simulink model "EdgeDetection"  (R2021a)
settings: Solver=VariableStepAuto  StartTime=0.0  StopTime=Ts_480p*2  RelTol=1e-3
InitFcn:
  | Ts = 1e-3;
  | Ts_240p = 402*324*Ts;
  | Ts_480p = 525*800*Ts;
undefined symbols (not defined in the file): gray, Rec, SDTV
libraries: hdlsllib x7, simulink x5, visionhdlio x2, visionhdlconversions x1, dspvision x1
settings Model: Creator=user  LastModifiedBy=user
settings OptimizationCC: BlockReduction=off  ConditionallyExecuteInputs=off  DefaultParameterBehavior=Inlined
settings DebuggingCC: AlgebraicLoopMsg=error
settings HardwareCC: ProdBitPerPointer=32  ProdBitPerSizeT=32  ProdBitPerPtrDiffT=32  ProdLargestAtomicFloat=None  ProdIntDivRoundTo=Undefined  ProdEndianess=Unspecified  ProdWordSize=32  ProdHWDeviceType=ASIC/FPGA->ASIC/FPGA  TargetBitPerPointer=64  TargetBitPerSizeT=64  TargetBitPerPtrDiffT=64  TargetLongLongMode=on  TargetIntDivRoundTo=Zero  TargetEndianess=LittleEndian  TargetWordSize=64  TargetHWDeviceType=Custom Processor->MATLAB Host Computer  ProdEqTarget=off

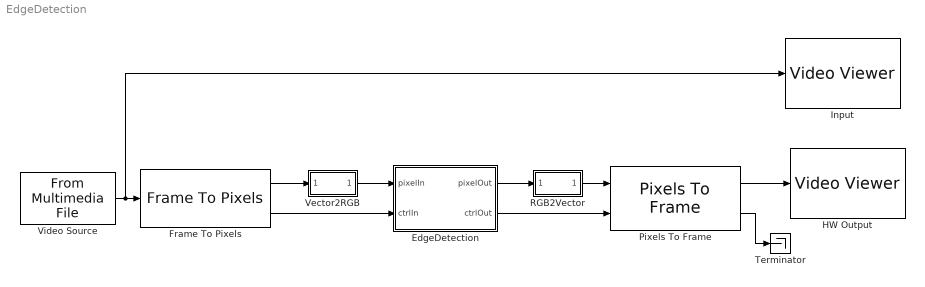
== system EdgeDetection ==
  EdgeDetection : Subsystem  TreatAsAtomicUnit=on
  Frame To Pixels : visionhdlio/Frame To Pixels  NumComponents=3  NumPixels=1  VideoFormat=480p  ActivePixelsPerLine=32  ActiveVideoLines=18  TotalPixelsPerLine=42  TotalVideoLines=28  StartingActiveLine=6  FrontPorch=5  SampleTime=0
      settings: SourceProductBaseCode=VT
  HW Output : VideoViewer  colormapValue=gray(256)  FigPos=[237 717 588 436]
  Input : VideoViewer  colormapValue=gray(256)  FigPos=[896 724 588 436]
  Pixels To Frame : visionhdlio/Pixels To Frame  NumComponents=3  NumPixels=1  VideoFormat=480p  ActivePixelsPerLine=32  ActiveVideoLines=18  TotalPixelsPerLine=42  TotalVideoLines=28
      settings: SourceProductBaseCode=VT
  RGB2Vector : Subsystem
  Terminator : Terminator
  Vector2RGB : Subsystem
  Video Source : dspvision/From Multimedia File  inputFilename=D:\Work\XilFPGAdev\Custom_IP_Cores\MathworksHDLCoder\testImages\engine_480p.bmp  readRange=[1 Inf]  loop=on  numPlays=inf  outputStreams=Video only  videoDataType=uint8  audioDataType=int16  inheritSampleTime=off  userDefinedSampleTime=Ts_480p  noAudioOutput=off  isIntensityVideo=off  fourcc=RGB  colorVideoFormat=One multidimensional signal  outputEOF=off  dataOrg=Column-major  audioFrameSize=1024  computeAudioFrameSize=off  outSamplingMode=Sample based
  wires:
  Vector2RGB/1(RGB) -> EdgeDetection/1(pixelIn)
  RGB2Vector/1(RGBVector) -> Pixels To Frame/1
  Frame To Pixels/1 -> Vector2RGB/1(RGBVector)
  Frame To Pixels/2 -> EdgeDetection/2(ctrlIn)
  Pixels To Frame/1 -> HW Output/1
  Pixels To Frame/2 -> Terminator/1
  Video Source/1 -> Input/1, Frame To Pixels/1
  EdgeDetection/1(pixelOut) -> RGB2Vector/1(RGB)
  EdgeDetection/2(ctrlOut) -> Pixels To Frame/2

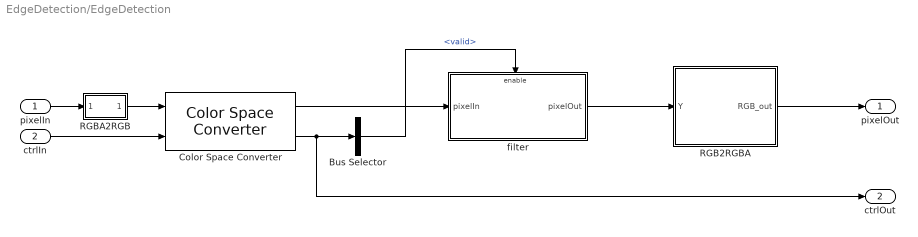
== system EdgeDetection/EdgeDetection ==
  pixelIn : Inport
  ctrlIn : Inport  Port=2
  Bus Selector : BusSelector  OutputSignals=valid
  Color Space Converter : visionhdlconversions/Color Space Converter  Conversion=RGB to intensity  ConversionStandard=Rec. 601 (SDTV)  ScanningStandard=1250/50/2:1  SimulateUsing=Code generation
      settings: SourceProductBaseCode=VT
  RGB2RGBA : MATLAB Function  TreatAsAtomicUnit=on
  RGBA2RGB : Subsystem
  filter : Subsystem
  pixelOut : Outport
  ctrlOut : Outport  Port=2  VectorParamsAs1DForOutWhenUnconnected=off
  wires:
  ctrlIn/1 -> Color Space Converter/2
  pixelIn/1 -> RGBA2RGB/1(RGBA)
  Color Space Converter/2 -> Bus Selector/1, ctrlOut/1
  RGBA2RGB/1(RGB) -> Color Space Converter/1
  RGB2RGBA/1(RGB_out) -> pixelOut/1
  Color Space Converter/1 -> filter/1(pixelIn)
  Bus Selector/1 -> filter/Enable  "<valid>"
  filter/1(pixelOut) -> RGB2RGBA/1(Y)

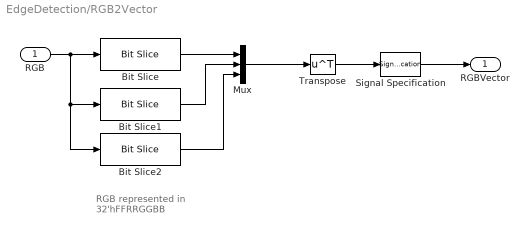
== system EdgeDetection/RGB2Vector ==
  note: RGB represented in
      | 32'hFFRRGGBB
  RGB : Inport
  Bit Slice : hdlsllib/Logic and Bit Operations/Bit Slice  lidx=23  ridx=16
      settings: SourceProductBaseCode=SL
  Bit Slice1 : hdlsllib/Logic and Bit Operations/Bit Slice  lidx=15  ridx=8
      settings: SourceProductBaseCode=SL
  Bit Slice2 : hdlsllib/Logic and Bit Operations/Bit Slice  lidx=7  ridx=0
      settings: SourceProductBaseCode=SL
  Mux : Mux  Inputs=3
  Signal Specification : SignalSpecification
  Transpose : Math  Operator=transpose  SignedPower=on  SaturateOnIntegerOverflow=on
  RGBVector : Outport  VectorParamsAs1DForOutWhenUnconnected=off
  wires:
  Mux/1 -> Transpose/1
  Bit Slice/1 -> Mux/1
  Bit Slice2/1 -> Mux/3
  Bit Slice1/1 -> Mux/2
  RGB/1 -> Bit Slice2/1, Bit Slice1/1, Bit Slice/1
  Transpose/1 -> Signal Specification/1
  Signal Specification/1 -> RGBVector/1

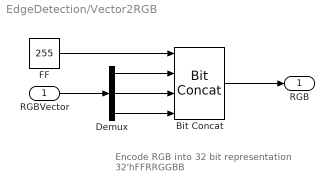
== system EdgeDetection/Vector2RGB ==
  note: Encode RGB into 32 bit representation
      | 32'hFFRRGGBB
  RGBVector : Inport
  Bit Concat : hdlsllib/Logic and Bit Operations/Bit Concat  numInputs=4
  Demux : Demux  Outputs=3
  FF : Constant  Value=255  OutDataTypeStr=uint8  SampleTime=Ts
  RGB : Outport  VectorParamsAs1DForOutWhenUnconnected=off
  wires:
  Bit Concat/1 -> RGB/1
  RGBVector/1 -> Demux/1
  FF/1 -> Bit Concat/1
  Demux/1 -> Bit Concat/2
  Demux/2 -> Bit Concat/3
  Demux/3 -> Bit Concat/4

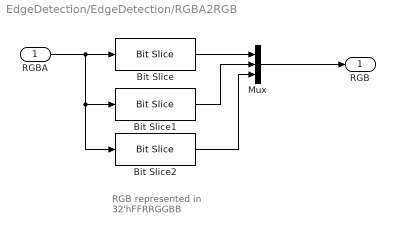
== system EdgeDetection/EdgeDetection/RGBA2RGB ==
  note: RGB represented in
      | 32'hFFRRGGBB
  RGBA : Inport
  Bit Slice : hdlsllib/Logic and Bit Operations/Bit Slice  lidx=23  ridx=16
      settings: SourceProductBaseCode=SL
  Bit Slice1 : hdlsllib/Logic and Bit Operations/Bit Slice  lidx=15  ridx=8
      settings: SourceProductBaseCode=SL
  Bit Slice2 : hdlsllib/Logic and Bit Operations/Bit Slice  lidx=7  ridx=0
      settings: SourceProductBaseCode=SL
  Mux : Mux  Inputs=3
  RGB : Outport  VectorParamsAs1DForOutWhenUnconnected=off
  wires:
  Bit Slice/1 -> Mux/1
  Bit Slice2/1 -> Mux/3
  Bit Slice1/1 -> Mux/2
  RGBA/1 -> Bit Slice2/1, Bit Slice1/1, Bit Slice/1
  Mux/1 -> RGB/1

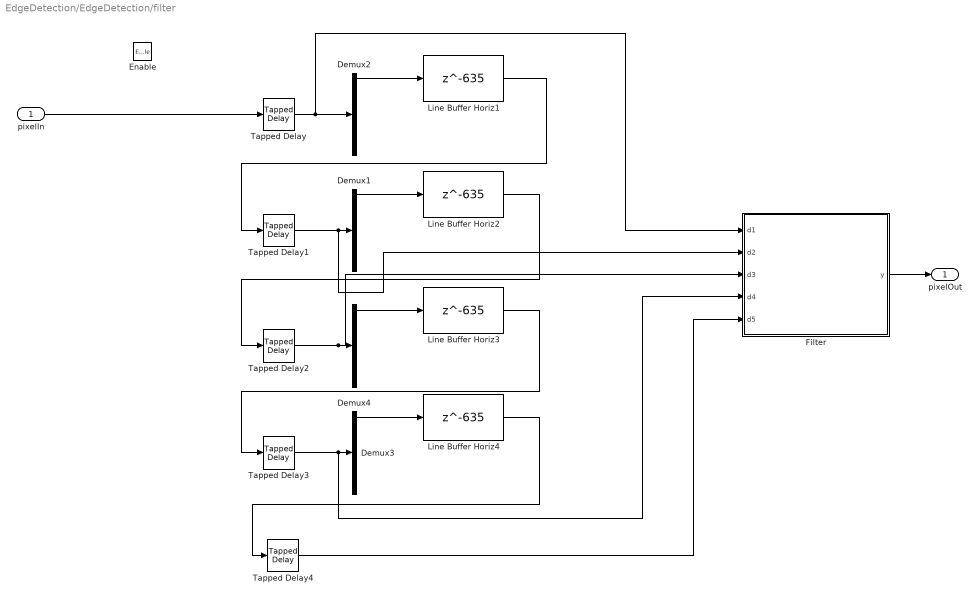
== system EdgeDetection/EdgeDetection/filter ==
  pixelIn : Inport
  Enable : EnablePort
  Demux{1..4} (4 alike) : Demux  Outputs=5
      settings: DisplayOption=none
  Filter : MATLAB Function  TreatAsAtomicUnit=on
  Line Buffer Horiz{1..4} (4 alike) : Delay  DelayLength=635  InitialCondition=0
  Tapped Delay{,1..4} (5 alike) : simulink/Discrete/Tapped Delay  vinit=0.0  samptime=-1  NumDelays=5  DelayOrder=Oldest  includeCurrent=on
  pixelOut : Outport  InitialOutput=0
  wires:
  Tapped Delay/1 -> Filter/1(d1), Demux2/1
  Demux2/1 -> Line Buffer Horiz1/1
  pixelIn/1 -> Tapped Delay/1
  Line Buffer Horiz1/1 -> Tapped Delay1/1
  Demux1/1 -> Line Buffer Horiz2/1
  Tapped Delay1/1 -> Filter/2(d2), Demux1/1
  Tapped Delay2/1 -> Filter/3(d3), Demux4/1
  Tapped Delay3/1 -> Filter/4(d4), Demux3/1
  Demux3/1 -> Line Buffer Horiz4/1
  Demux4/1 -> Line Buffer Horiz3/1
  Line Buffer Horiz2/1 -> Tapped Delay2/1
  Line Buffer Horiz3/1 -> Tapped Delay3/1
  Line Buffer Horiz4/1 -> Tapped Delay4/1
  Tapped Delay4/1 -> Filter/5(d5)
  Filter/1(y) -> pixelOut/1

== matlab function EdgeDetection/RGB2RGBA ==
  data: Y input; RGB_out output
function RGB_out = Concat_Sig(Y)
% 32'hAARRBBGG
Y = Y *2;
Rd = fi(Y, 0, 8, 0);
Gr = fi(Y, 0, 8, 0);
Bl = fi(Y, 0, 8, 0);
AA = fi(255, 0, 8, 0);
RGB_out = bitconcat(AA,Rd,Gr,Bl);

== matlab function EdgeDetection/filter/Filter ==
  data: d1 input; y output; d2 input; d3 input; d4 input; d5 input
function y = fcn(d1,d2,d3,d4,d5)
d = [d1,d2,d3,d4,d5]';
d = fi(d,0,8,0);
% s = sum(sum(d))/fi(25,0,5,0);

dx = d(3,1) + fi(2,0,2,0)*d(3,2) - fi(2,0,2,0)*d(3,4) - d(3,5);
dy = d(1,3) + fi(2,0,2,0)*d(2,3) - fi(2,0,2,0)*d(4,3) - d(5,3);
s = (abs(dx) + abs(dy))/fi(2,0,2,0);

y = fi(s, 0, 8, 0);
